simulink model "CarController"  (R2021a)
settings: Solver=FixedStepAuto  StartTime=0.0  StopTime=inf  FixedStep=0.01  RelTol=1e-3  EnableMultiTasking=on
model workspace (MAT data in the model file):
  sample_time = 0.01
libraries: dspnetwork x8
settings Model: xpc_rtwmakecfg_data=_xpcnblib__xpcetherlib__xpcether8255xlib__xpcetherGbElib__xpciplib_  Creator=rudol  LastModifiedBy=DHEEPAK
settings SolverCC: AlgebraicLoopSolver=TrustRegion
settings DataIOCC: LimitDataPoints=on  SaveFormat=Array  ReturnWorkspaceOutputs=off
settings OptimizationCC: LifeSpan=inf
settings DebuggingCC: SFUnexpectedBacktrackingDiag=warning  SFNoUnconditionalDefaultTransitionDiag=warning  SFExecutionAtInitializationDiag=none  SFMachineParentedDataDiag=warning  ArithmeticOperatorsInVariantConditions=warning
settings HardwareCC: ProdBitPerPointer=32  ProdBitPerSizeT=32  ProdBitPerPtrDiffT=32  ProdLargestAtomicFloat=None  ProdIntDivRoundTo=Undefined  ProdEndianess=Unspecified  ProdWordSize=32  ProdHWDeviceType=32-bit Generic
settings ModelReferenceCC: EnableRefExpFcnMdlSchedulingChecks=off  PropagateSignalLabelsOutOfModel=off
settings SFSimCC: SimUseLocalCustomCode=off  CustomCodeUndefinedFunction=UseInterfaceOnly
settings RTWCC: RTWUseLocalCustomCode=off
settings CodeAppCC: StateflowObjectComments=on
settings GRTTargetCC: TargetLangStandard=C89/C90 (ANSI)
settings ConfigComp: CovMetricSettings=dw  CovSaveCumulativeToWorkspaceVar=on  CovSaveSingleToWorkspaceVar=on  CovExternalEMLEnable=off

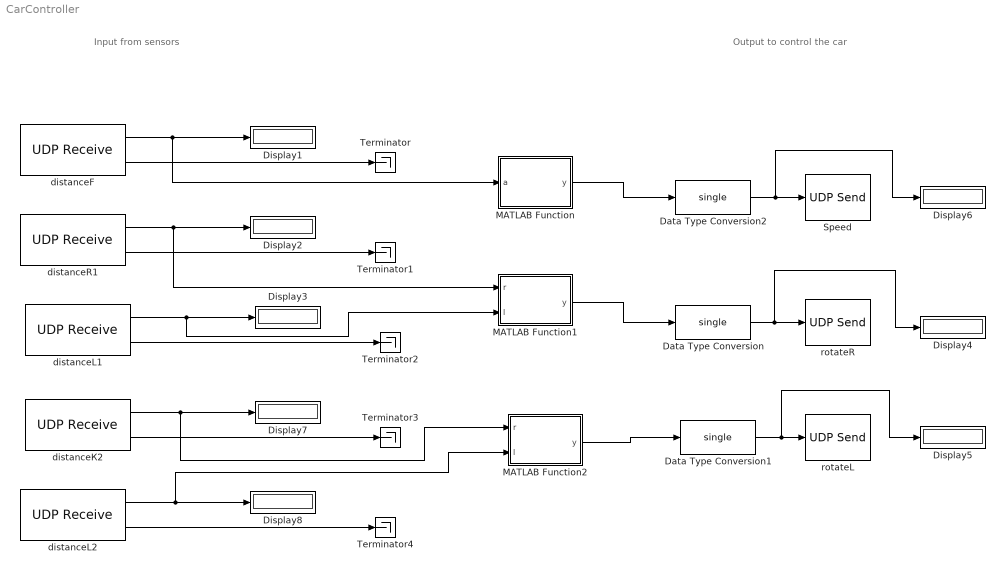
== system CarController ==
  note: Input from sensors
  note: Output to control the car
  Data Type Conversion : DataTypeConversion  OutDataTypeStr=single
  Data Type Conversion1 : DataTypeConversion  OutDataTypeStr=single
  Data Type Conversion2 : DataTypeConversion  OutDataTypeStr=single
  Display{1..8} (8 alike) : Display
  MATLAB Function : MATLAB Function  TreatAsAtomicUnit=on
  MATLAB Function1 : MATLAB Function  TreatAsAtomicUnit=on
  MATLAB Function2 : MATLAB Function  TreatAsAtomicUnit=on
  Speed : dspnetwork/UDP Send  remoteURL='127.0.0.1'  remotePort=9900  localURL='0.0.0.0'  localPortSource=Automatically determine  localPort=-1  sendBufferSize=8192  sampletime=-1  blockPlatform=[]  separateLengthPort=0
  Terminator{,1..4} (5 alike) : Terminator
  distanceF : dspnetwork/UDP Receive  localURL='0.0.0.0'  localPort=10  remoteURL='0.0.0.0'  remotePort=-1  recvBufferSize=8192  dims=1  signalDatatype=single  isComplex=off  isVarSize=off  showBlockingTime=off  blockingTime=0  sampletime=sample_time  blockPlatform=[]
  distanceL1 : dspnetwork/UDP Receive  localURL='0.0.0.0'  localPort=12  remoteURL='0.0.0.0'  remotePort=-1  recvBufferSize=8192  dims=1  signalDatatype=single  isComplex=off  isVarSize=off  showBlockingTime=off  blockingTime=0  sampletime=sample_time  blockPlatform=[]
  distanceL2 : dspnetwork/UDP Receive  localURL='0.0.0.0'  localPort=14  remoteURL='0.0.0.0'  remotePort=-1  recvBufferSize=8192  dims=1  signalDatatype=single  isComplex=off  isVarSize=off  showBlockingTime=off  blockingTime=0  sampletime=sample_time  blockPlatform=[]
  distanceR1 : dspnetwork/UDP Receive  localURL='0.0.0.0'  localPort=11  remoteURL='0.0.0.0'  remotePort=-1  recvBufferSize=8192  dims=1  signalDatatype=single  isComplex=off  isVarSize=off  showBlockingTime=off  blockingTime=0  sampletime=sample_time  blockPlatform=[]
  distanceК2 : dspnetwork/UDP Receive  localURL='0.0.0.0'  localPort=13  remoteURL='0.0.0.0'  remotePort=-1  recvBufferSize=8192  dims=1  signalDatatype=single  isComplex=off  isVarSize=off  showBlockingTime=off  blockingTime=0  sampletime=sample_time  blockPlatform=[]
  rotateL : dspnetwork/UDP Send  remoteURL='127.0.0.1'  remotePort=120  localURL='0.0.0.0'  localPortSource=Automatically determine  localPort=-1  sendBufferSize=8192  sampletime=-1  blockPlatform=[]  separateLengthPort=0
  rotateR : dspnetwork/UDP Send  remoteURL='127.0.0.1'  remotePort=130  localURL='0.0.0.0'  localPortSource=Automatically determine  localPort=-1  sendBufferSize=8192  sampletime=-1  blockPlatform=[]  separateLengthPort=0
  wires:
  Data Type Conversion1/1 -> rotateL/1, Display5/1
  Data Type Conversion/1 -> Display4/1, rotateR/1
  Data Type Conversion2/1 -> Speed/1, Display6/1
  distanceL2/1 -> MATLAB Function2/2(l), Display8/1
  distanceR1/2 -> Terminator1/1
  distanceF/2 -> Terminator/1
  distanceL1/2 -> Terminator2/1
  distanceК2/2 -> Terminator3/1
  distanceL2/2 -> Terminator4/1
  distanceF/1 -> MATLAB Function/1(a), Display1/1
  MATLAB Function/1(y) -> Data Type Conversion2/1
  distanceК2/1 -> MATLAB Function2/1(r), Display7/1
  distanceL1/1 -> MATLAB Function1/2(l), Display3/1
  distanceR1/1 -> MATLAB Function1/1(r), Display2/1
  MATLAB Function2/1(y) -> Data Type Conversion1/1
  MATLAB Function1/1(y) -> Data Type Conversion/1

== matlab function CarController/MATLAB Function ==
  data: a input; y output
function y = fcn(a)
    if a < 20
        a=a-(0.2*a); 
    end
    y = a;
end

== matlab function CarController/MATLAB Function2 ==
  data: r input; y output; l input
function y = fcn(r,l)

m = (r+l)/2;
buffer = 1;  

if abs(r-m) > buffer
    z = single(r-m);
    y = -z;
elseif l-m > buffer
     z = single(l-m);
     y = -z;
else
    y =single(0);

end

% function y = fcn(a,b)
% if a < 5
%     a = a-(a*0.2);
% end
% y = a;
% end

== matlab function CarController/MATLAB Function1 ==
  data: r input; y output; l input
function y = fcn(r,l)

m = (r+l)/2;
buffer = 1;  

if abs(r-m) > buffer
    z = single(r-m);
    y = -z;
elseif l-m > buffer
     z = single(l-m);
     y = -z;
else
    y =single(0);

end
